simulink model "dyn_nielin_mod_ciagly"  (R2014b)
settings: Solver=ode45  StartTime=0.0  StopTime=tkonc  RelTol=1e-3
undefined symbols (not defined in the file): a1, a2, a3, a4, K, T1, T2, x0
settings Model: Creator=Konrad  LastModifiedBy=Konrad

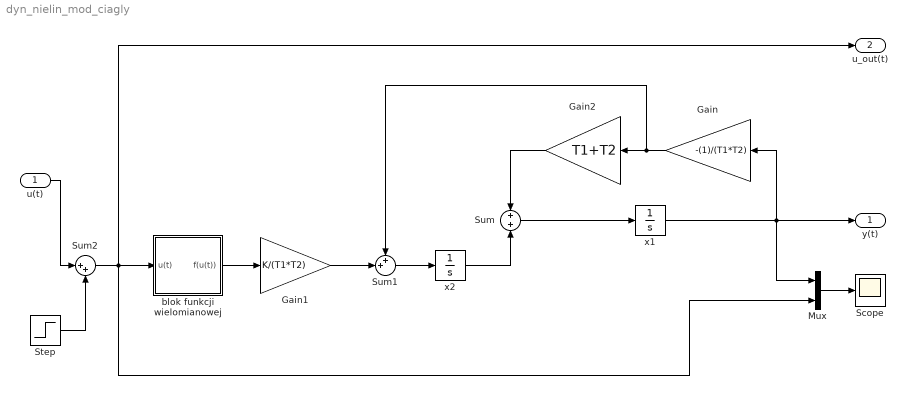
== system dyn_nielin_mod_ciagly ==
  u(t) : Inport
  Gain : Gain  Gain=-(1)/(T1*T2)
  Gain1 : Gain  Gain=K/(T1*T2)
  Gain2 : Gain  Gain=T1+T2
  Mux : Mux  Inputs=2
  Scope : Scope
  Step : Step  SampleTime=0
  Sum : Sum
  Sum1 : Sum  Inputs=++|
  Sum2 : Sum  Inputs=|++
  blok funkcji wielomianowej : Subsystem
  x1 : Integrator  InitialCondition=x0(1)  ContinuousStateAttributes='x1'
  x2 : Integrator  InitialCondition=x0(2)  ContinuousStateAttributes='x2'
  y(t) : Outport
  u_out(t) : Outport  Port=2
  wires:
  x1/1 -> y(t)/1, Gain/1, Mux/1
  Sum/1 -> x1/1
  x2/1 -> Sum/2
  Gain/1 -> Gain2/1, Sum1/1
  Gain2/1 -> Sum/1
  Sum1/1 -> x2/1
  Gain1/1 -> Sum1/2
  blok funkcji wielomianowej/1(f(u(t))) -> Gain1/1
  Sum2/1 -> u_out(t)/1, Mux/2, blok funkcji wielomianowej/1(u(t))
  Mux/1 -> Scope/1
  Step/1 -> Sum2/2
  u(t)/1 -> Sum2/1

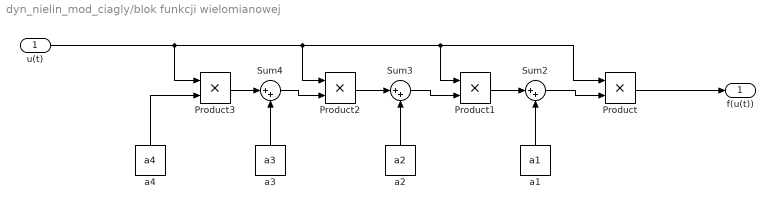
== system dyn_nielin_mod_ciagly/blok funkcji wielomianowej ==
  u(t) : Inport
  Product{,1..3} (4 alike) : Product
  Sum2 : Sum  Inputs=|++
  Sum3 : Sum  Inputs=|++
  Sum4 : Sum  Inputs=|++
  a1 : Constant  Value=a1
  a2 : Constant  Value=a2
  a3 : Constant  Value=a3
  a4 : Constant  Value=a4
  f(u(t)) : Outport
  wires:
  u(t)/1 -> Product/1, Product1/1, Product2/1, Product3/1
  Product1/1 -> Sum2/1
  Product2/1 -> Sum3/1
  Sum2/1 -> Product/2
  Product/1 -> f(u(t))/1
  Product3/1 -> Sum4/1
  a1/1 -> Sum2/2
  a2/1 -> Sum3/2
  Sum3/1 -> Product1/2
  a3/1 -> Sum4/2
  Sum4/1 -> Product2/2
  a4/1 -> Product3/2
